simulink model "kamerol"  (R2021b)
settings: Solver=VariableStepAuto  StartTime=0.0  StopTime=10.0  RelTol=1e-3
undefined symbols (not defined in the file): admireDB
libraries: simulink_extras x104, simulink x24, sharedutil x1
(part 11 of 14)

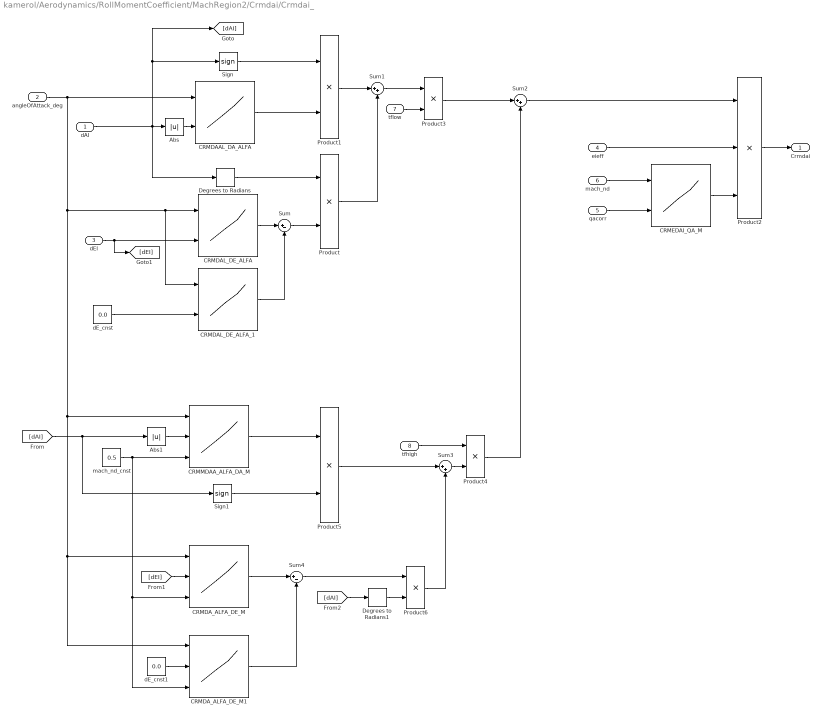
== system kamerol/Aerodynamics/RollMomentCoefficient/MachRegion2/Crmdai/Crmdai_ ==
  dAI : Inport
  angleOfAttack_deg : Inport  Port=2
  dEI : Inport  Port=3
  eieff : Inport  Port=4
  qacorr : Inport  Port=5
  mach_nd : Inport  Port=6
  tflow : Inport  Port=7
  tfhigh : Inport  Port=8
  Abs : Abs
  Abs1 : Abs
  CRMDAAL_DA_ALFA : Lookup_n-D  BreakpointsForDimension1=admireDB.aerodata_asym_ext.CRMDAAL.breakpoints.ALFA  BreakpointsForDimension2=admireDB.aerodata_asym_ext.CRMDAAL.breakpoints.DA  BreakpointsForDimension3=[5, 7]  Table=admireDB.aerodata_asym_ext.CRMDAAL.newTable  ExtrapMethod=Clip  InternalRulePriority=Speed  RndMeth=Simplest  InputSameDT=on
      settings: InputPortMap=u0,u1
  CRMDAL_DE_ALFA : Lookup_n-D  BreakpointsForDimension1=admireDB.aerodata_asym_ext.CRMDAL.breakpoints.ALFA  BreakpointsForDimension2=admireDB.aerodata_asym_ext.CRMDAL.breakpoints.DE  BreakpointsForDimension3=[5, 7]  Table=admireDB.aerodata_asym_ext.CRMDAL.newTable  ExtrapMethod=Clip  InternalRulePriority=Speed  RndMeth=Simplest  InputSameDT=on
      settings: InputPortMap=u0,u1
  CRMDAL_DE_ALFA_1 : Lookup_n-D  BreakpointsForDimension1=admireDB.aerodata_asym_ext.CRMDAL.breakpoints.ALFA  BreakpointsForDimension2=admireDB.aerodata_asym_ext.CRMDAL.breakpoints.DE  BreakpointsForDimension3=[5, 7]  Table=admireDB.aerodata_asym_ext.CRMDAL.newTable  ExtrapMethod=Clip  InternalRulePriority=Speed  RndMeth=Simplest  InputSameDT=on
      settings: InputPortMap=u0,u1
  CRMDA_ALFA_DE_M : Lookup_n-D  NumberOfTableDimensions=3  BreakpointsForDimension1=admireDB.aerodata_asym_ext.CRMDA.breakpoints.ALFA  BreakpointsForDimension2=admireDB.aerodata_asym_ext.CRMDA.breakpoints.DE  BreakpointsForDimension3=admireDB.aerodata_asym_ext.CRMDA.breakpoints.M  Table=admireDB.aerodata_asym_ext.CRMDA.newTable  ExtrapMethod=Clip  InternalRulePriority=Speed  RndMeth=Simplest  InputSameDT=on
      settings: InputPortMap=u0,u1,u2
  CRMDA_ALFA_DE_M1 : Lookup_n-D  NumberOfTableDimensions=3  BreakpointsForDimension1=admireDB.aerodata_asym_ext.CRMDA.breakpoints.ALFA  BreakpointsForDimension2=admireDB.aerodata_asym_ext.CRMDA.breakpoints.DE  BreakpointsForDimension3=admireDB.aerodata_asym_ext.CRMDA.breakpoints.M  Table=admireDB.aerodata_asym_ext.CRMDA.newTable  ExtrapMethod=Clip  InternalRulePriority=Speed  RndMeth=Simplest  InputSameDT=on
      settings: InputPortMap=u0,u1,u2
  CRMEDAI_QA_M : Lookup_n-D  BreakpointsForDimension1=admireDB.aerodata_asym_ext.CRMEDAI.breakpoints.M  BreakpointsForDimension2=admireDB.aerodata_asym_ext.CRMEDAI.breakpoints.QA  BreakpointsForDimension3=[5, 7]  Table=admireDB.aerodata_asym_ext.CRMEDAI.newTable  ExtrapMethod=Clip  InternalRulePriority=Speed  RndMeth=Simplest  InputSameDT=on
      settings: InputPortMap=u0,u1
  CRMMDAA_ALFA_DA_M : Lookup_n-D  NumberOfTableDimensions=3  BreakpointsForDimension1=admireDB.aerodata_asym_ext.CRMMDAA.breakpoints.ALFA  BreakpointsForDimension2=admireDB.aerodata_asym_ext.CRMMDAA.breakpoints.DA  BreakpointsForDimension3=admireDB.aerodata_asym_ext.CRMMDAA.breakpoints.M  Table=admireDB.aerodata_asym_ext.CRMMDAA.newTable  ExtrapMethod=Clip  InternalRulePriority=Speed  RndMeth=Simplest  InputSameDT=on
      settings: InputPortMap=u0,u1,u2
  Degrees to Radians : simulink_extras/Transformations/Degrees to Radians
  Degrees to Radians1 : simulink_extras/Transformations/Degrees to Radians
  Product{,1,3..4,6} (5 alike) : Product
  Product2 : Product  Inputs=3
  Product5 : Product  Inputs=**
  Sign : Signum
  Sign1 : Signum
  Sum : Sum  Inputs=|+-
  Sum1 : Sum  Inputs=|++
  Sum2 : Sum  Inputs=|++
  Sum3 : Sum  Inputs=|++
  Sum4 : Sum  Inputs=|+-
  dE_cnst : Constant  Value=0.0
  dE_cnst1 : Constant  Value=0.0
  mach_nd_cnst : Constant  Value=0.5
  Crmdai : Outport
  wires:
  Sum3/1 -> Product4/2
  Product6/1 -> Sum3/2
  [dAI] -> Degrees to Radians1/1
  Degrees to Radians1/1 -> Product6/2
  Sum4/1 -> Product6/1
  CRMDA_ALFA_DE_M1/1 -> Sum4/2
  CRMDA_ALFA_DE_M/1 -> Sum4/1
  dE_cnst1/1 -> CRMDA_ALFA_DE_M1/2
  [dEI] -> CRMDA_ALFA_DE_M/2
  mach_nd_cnst/1 -> CRMDA_ALFA_DE_M/3, CRMDA_ALFA_DE_M1/3, CRMMDAA_ALFA_DA_M/3
  Product5/1 -> Sum3/1
  Abs1/1 -> CRMMDAA_ALFA_DA_M/2
  CRMMDAA_ALFA_DA_M/1 -> Product5/1
  [dAI] -> Sign1/1, Abs1/1
  Sign1/1 -> Product5/2
  angleOfAttack_deg/1 -> CRMDAAL_DA_ALFA/1, CRMDAL_DE_ALFA/1, CRMDAL_DE_ALFA_1/1, CRMMDAA_ALFA_DA_M/1, CRMDA_ALFA_DE_M1/1, CRMDA_ALFA_DE_M/1
  Product4/1 -> Sum2/2
  Product3/1 -> Sum2/1
  tfhigh/1 -> Product4/1
  Sum2/1 -> Product2/1
  tflow/1 -> Product3/2
  Product2/1 -> Crmdai/1
  dAI/1 -> Sign/1, [dAI], Abs/1, Degrees to Radians/1
  Abs/1 -> CRMDAAL_DA_ALFA/2
  dE_cnst/1 -> CRMDAL_DE_ALFA_1/2
  dEI/1 -> [dEI], CRMDAL_DE_ALFA/2
  CRMDAL_DE_ALFA/1 -> Sum/1
  CRMDAL_DE_ALFA_1/1 -> Sum/2
  Sum/1 -> Product/2
  Degrees to Radians/1 -> Product/1
  CRMDAAL_DA_ALFA/1 -> Product1/2
  Sign/1 -> Product1/1
  Product1/1 -> Sum1/1
  Product/1 -> Sum1/2
  Sum1/1 -> Product3/1
  eieff/1 -> Product2/2
  qacorr/1 -> CRMEDAI_QA_M/2
  mach_nd/1 -> CRMEDAI_QA_M/1
  CRMEDAI_QA_M/1 -> Product2/3

== system kamerol/Aerodynamics/RollMomentCoefficient/MachRegion2/Crmdaib/Crmdaib_ ==
  angleOfAttack_deg : Inport
  dAI : Inport  Port=2
  angleOfSideslip_deg : Inport  Port=3
  eieff : Inport  Port=4
  tflow : Inport  Port=5
  Abs : Abs
  Abs1 : Abs
  Abs2 : Abs
  CRMDABAL_ALFA : Lookup_n-D  NumberOfTableDimensions=1  BreakpointsForDimension1=admireDB.aerodata_asym_ext.CRMDABAL.breakpoints.ALFA  BreakpointsForDimension3=[5, 7]  Table=admireDB.aerodata_asym_ext.CRMDABAL.newTable  ExtrapMethod=Clip  InternalRulePriority=Speed  RndMeth=Simplest  InputSameDT=on
  Constant : Constant  Value=1/30
  Constant1 : Constant  Value=1/20
  Product : Product  Inputs=*******
  Crmdaib : Outport
  wires:
  tflow/1 -> Product/7
  Product/1 -> Crmdaib/1
  angleOfAttack_deg/1 -> Abs/1
  CRMDABAL_ALFA/1 -> Product/1
  dAI/1 -> Abs1/1
  Abs/1 -> CRMDABAL_ALFA/1
  Abs1/1 -> Product/2
  Constant/1 -> Product/3
  angleOfSideslip_deg/1 -> Abs2/1
  Constant1/1 -> Product/5
  Abs2/1 -> Product/4
  eieff/1 -> Product/6

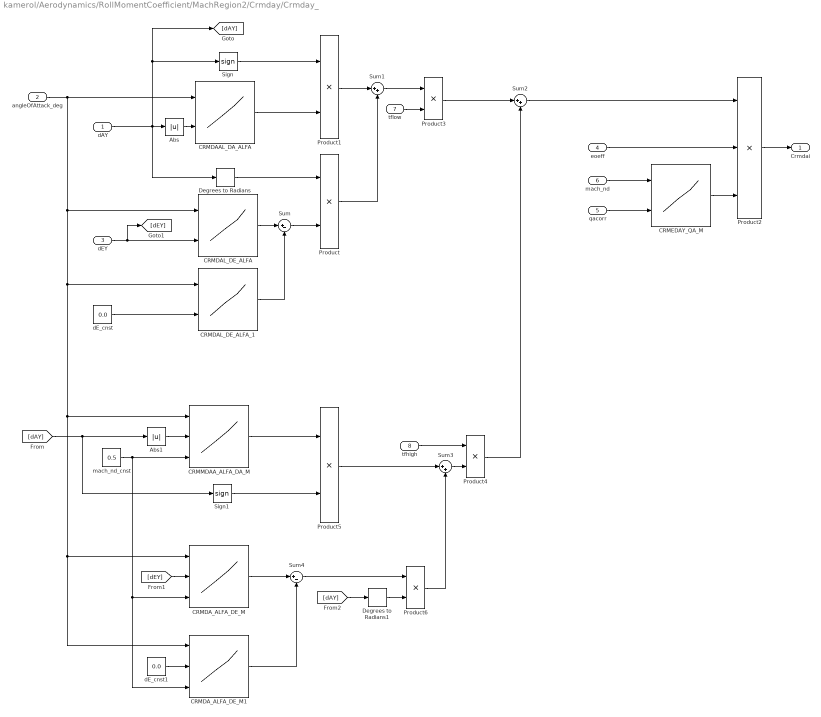
== system kamerol/Aerodynamics/RollMomentCoefficient/MachRegion2/Crmday/Crmday_ ==
  dAY : Inport
  angleOfAttack_deg : Inport  Port=2
  dEY : Inport  Port=3
  eoeff : Inport  Port=4
  qacorr : Inport  Port=5
  mach_nd : Inport  Port=6
  tflow : Inport  Port=7
  tfhigh : Inport  Port=8
  Abs : Abs
  Abs1 : Abs
  CRMDAAL_DA_ALFA : Lookup_n-D  BreakpointsForDimension1=admireDB.aerodata_asym_ext.CRMDAAL.breakpoints.ALFA  BreakpointsForDimension2=admireDB.aerodata_asym_ext.CRMDAAL.breakpoints.DA  BreakpointsForDimension3=[5, 7]  Table=admireDB.aerodata_asym_ext.CRMDAAL.newTable  ExtrapMethod=Clip  InternalRulePriority=Speed  RndMeth=Simplest  InputSameDT=on
      settings: InputPortMap=u0,u1
  CRMDAL_DE_ALFA : Lookup_n-D  BreakpointsForDimension1=admireDB.aerodata_asym_ext.CRMDAL.breakpoints.ALFA  BreakpointsForDimension2=admireDB.aerodata_asym_ext.CRMDAL.breakpoints.DE  BreakpointsForDimension3=[5, 7]  Table=admireDB.aerodata_asym_ext.CRMDAL.newTable  ExtrapMethod=Clip  InternalRulePriority=Speed  RndMeth=Simplest  InputSameDT=on
      settings: InputPortMap=u0,u1
  CRMDAL_DE_ALFA_1 : Lookup_n-D  BreakpointsForDimension1=admireDB.aerodata_asym_ext.CRMDAL.breakpoints.ALFA  BreakpointsForDimension2=admireDB.aerodata_asym_ext.CRMDAL.breakpoints.DE  BreakpointsForDimension3=[5, 7]  Table=admireDB.aerodata_asym_ext.CRMDAL.newTable  ExtrapMethod=Clip  InternalRulePriority=Speed  RndMeth=Simplest  InputSameDT=on
      settings: InputPortMap=u0,u1
  CRMDA_ALFA_DE_M : Lookup_n-D  NumberOfTableDimensions=3  BreakpointsForDimension1=admireDB.aerodata_asym_ext.CRMDA.breakpoints.ALFA  BreakpointsForDimension2=admireDB.aerodata_asym_ext.CRMDA.breakpoints.DE  BreakpointsForDimension3=admireDB.aerodata_asym_ext.CRMDA.breakpoints.M  Table=admireDB.aerodata_asym_ext.CRMDA.newTable  ExtrapMethod=Clip  InternalRulePriority=Speed  RndMeth=Simplest  InputSameDT=on
      settings: InputPortMap=u0,u1,u2
  CRMDA_ALFA_DE_M1 : Lookup_n-D  NumberOfTableDimensions=3  BreakpointsForDimension1=admireDB.aerodata_asym_ext.CRMDA.breakpoints.ALFA  BreakpointsForDimension2=admireDB.aerodata_asym_ext.CRMDA.breakpoints.DE  BreakpointsForDimension3=admireDB.aerodata_asym_ext.CRMDA.breakpoints.M  Table=admireDB.aerodata_asym_ext.CRMDA.newTable  ExtrapMethod=Clip  InternalRulePriority=Speed  RndMeth=Simplest  InputSameDT=on
      settings: InputPortMap=u0,u1,u2
  CRMEDAY_QA_M : Lookup_n-D  BreakpointsForDimension1=admireDB.aerodata_asym_ext.CRMEDAY.breakpoints.M  BreakpointsForDimension2=admireDB.aerodata_asym_ext.CRMEDAY.breakpoints.QA  BreakpointsForDimension3=[5, 7]  Table=admireDB.aerodata_asym_ext.CRMEDAY.newTable  ExtrapMethod=Clip  InternalRulePriority=Speed  RndMeth=Simplest  InputSameDT=on
      settings: InputPortMap=u0,u1
  CRMMDAA_ALFA_DA_M : Lookup_n-D  NumberOfTableDimensions=3  BreakpointsForDimension1=admireDB.aerodata_asym_ext.CRMMDAA.breakpoints.ALFA  BreakpointsForDimension2=admireDB.aerodata_asym_ext.CRMMDAA.breakpoints.DA  BreakpointsForDimension3=admireDB.aerodata_asym_ext.CRMMDAA.breakpoints.M  Table=admireDB.aerodata_asym_ext.CRMMDAA.newTable  ExtrapMethod=Clip  InternalRulePriority=Speed  RndMeth=Simplest  InputSameDT=on
      settings: InputPortMap=u0,u1,u2
  Degrees to Radians : simulink_extras/Transformations/Degrees to Radians
  Degrees to Radians1 : simulink_extras/Transformations/Degrees to Radians
  Product{,1,3..4,6} (5 alike) : Product
  Product2 : Product  Inputs=3
  Product5 : Product  Inputs=**
  Sign : Signum
  Sign1 : Signum
  Sum : Sum  Inputs=|+-
  Sum1 : Sum  Inputs=|++
  Sum2 : Sum  Inputs=|++
  Sum3 : Sum  Inputs=|++
  Sum4 : Sum  Inputs=|+-
  dE_cnst : Constant  Value=0.0
  dE_cnst1 : Constant  Value=0.0
  mach_nd_cnst : Constant  Value=0.5
  Crmdai : Outport
  wires:
  Sum3/1 -> Product4/2
  Product6/1 -> Sum3/2
  [dAY] -> Degrees to Radians1/1
  Degrees to Radians1/1 -> Product6/2
  Sum4/1 -> Product6/1
  CRMDA_ALFA_DE_M1/1 -> Sum4/2
  CRMDA_ALFA_DE_M/1 -> Sum4/1
  dE_cnst1/1 -> CRMDA_ALFA_DE_M1/2
  [dEY] -> CRMDA_ALFA_DE_M/2
  mach_nd_cnst/1 -> CRMDA_ALFA_DE_M/3, CRMDA_ALFA_DE_M1/3, CRMMDAA_ALFA_DA_M/3
  Product5/1 -> Sum3/1
  Abs1/1 -> CRMMDAA_ALFA_DA_M/2
  CRMMDAA_ALFA_DA_M/1 -> Product5/1
  [dAY] -> Sign1/1, Abs1/1
  Sign1/1 -> Product5/2
  angleOfAttack_deg/1 -> CRMDAAL_DA_ALFA/1, CRMDAL_DE_ALFA/1, CRMMDAA_ALFA_DA_M/1, CRMDA_ALFA_DE_M1/1, CRMDA_ALFA_DE_M/1, CRMDAL_DE_ALFA_1/1
  Product4/1 -> Sum2/2
  Product3/1 -> Sum2/1
  tfhigh/1 -> Product4/1
  Sum2/1 -> Product2/1
  tflow/1 -> Product3/2
  Product2/1 -> Crmdai/1
  dAY/1 -> Sign/1, [dAY], Abs/1, Degrees to Radians/1
  Abs/1 -> CRMDAAL_DA_ALFA/2
  dE_cnst/1 -> CRMDAL_DE_ALFA_1/2
  dEY/1 -> CRMDAL_DE_ALFA/2, [dEY]
  CRMDAL_DE_ALFA/1 -> Sum/1
  CRMDAL_DE_ALFA_1/1 -> Sum/2
  Sum/1 -> Product/2
  Degrees to Radians/1 -> Product/1
  CRMDAAL_DA_ALFA/1 -> Product1/2
  Sign/1 -> Product1/1
  Product1/1 -> Sum1/1
  Product/1 -> Sum1/2
  Sum1/1 -> Product3/1
  eoeff/1 -> Product2/2
  qacorr/1 -> CRMEDAY_QA_M/2
  mach_nd/1 -> CRMEDAY_QA_M/1
  CRMEDAY_QA_M/1 -> Product2/3

== system kamerol/Aerodynamics/RollMomentCoefficient/MachRegion2/Crmdayb/Crmdayb_ ==
  angleOfAttack_deg : Inport
  dAY : Inport  Port=2
  angleOfSideslip_deg : Inport  Port=3
  eoeff : Inport  Port=4
  tflow : Inport  Port=5
  Abs : Abs
  Abs1 : Abs
  Abs2 : Abs
  CRMDABAL_ALFA : Lookup_n-D  NumberOfTableDimensions=1  BreakpointsForDimension1=admireDB.aerodata_asym_ext.CRMDABAL.breakpoints.ALFA  BreakpointsForDimension3=[5, 7]  Table=admireDB.aerodata_asym_ext.CRMDABAL.newTable  ExtrapMethod=Clip  InternalRulePriority=Speed  RndMeth=Simplest  InputSameDT=on
  Constant : Constant  Value=1/30
  Constant1 : Constant  Value=1/20
  Product : Product  Inputs=*******
  Crmdayb : Outport
  wires:
  tflow/1 -> Product/7
  eoeff/1 -> Product/6
  Abs2/1 -> Product/4
  Constant1/1 -> Product/5
  angleOfSideslip_deg/1 -> Abs2/1
  Constant/1 -> Product/3
  Abs1/1 -> Product/2
  Abs/1 -> CRMDABAL_ALFA/1
  dAY/1 -> Abs1/1
  CRMDABAL_ALFA/1 -> Product/1
  angleOfAttack_deg/1 -> Abs/1
  Product/1 -> Crmdayb/1

== system kamerol/Aerodynamics/RollMomentCoefficient/MachRegion2/Crmdna/Crmdna_ ==
  dNE : Inport
  angleOfAttack_deg : Inport  Port=2
  tflow : Inport  Port=3
  tfhigh : Inport  Port=4
  dNA : Inport  Port=5
  CRMDNAAL_DNE_ALFA : Lookup_n-D  BreakpointsForDimension1=admireDB.aerodata_asym_ext.CRMDNAAL.breakpoints.ALFA  BreakpointsForDimension2=admireDB.aerodata_asym_ext.CRMDNAAL.breakpoints.DNE  BreakpointsForDimension3=[5, 7]  Table=admireDB.aerodata_asym_ext.CRMDNAAL.newTable  ExtrapMethod=Clip  InternalRulePriority=Speed  RndMeth=Simplest  InputSameDT=on
      settings: InputPortMap=u0,u1
  CRMDNAAM_ALFA_M : Lookup_n-D  BreakpointsForDimension1=admireDB.aerodata_asym_ext.CRMDNAAM.breakpoints.M  BreakpointsForDimension2=admireDB.aerodata_asym_ext.CRMDNAAM.breakpoints.ALFA  BreakpointsForDimension3=[5, 7]  Table=admireDB.aerodata_asym_ext.CRMDNAAM.newTable  ExtrapMethod=Clip  InternalRulePriority=Speed  RndMeth=Simplest  InputSameDT=on
      settings: InputPortMap=u0,u1
  Degrees to Radians : simulink_extras/Transformations/Degrees to Radians
  Product : Product  Inputs=**
  Product1 : Product
  Product2 : Product  Inputs=**
  Sum : Sum  Inputs=|++
  mach_nd_cnst : Constant  Value=0.5
  Crmdna : Outport
  wires:
  Sum/1 -> Product/1
  Product2/1 -> Sum/2
  Product1/1 -> Sum/1
  CRMDNAAM_ALFA_M/1 -> Product2/1
  tfhigh/1 -> Product2/2
  mach_nd_cnst/1 -> CRMDNAAM_ALFA_M/1
  tflow/1 -> Product1/2
  Product/1 -> Crmdna/1
  angleOfAttack_deg/1 -> CRMDNAAL_DNE_ALFA/1, CRMDNAAM_ALFA_M/2
  dNE/1 -> CRMDNAAL_DNE_ALFA/2
  dNA/1 -> Degrees to Radians/1
  CRMDNAAL_DNE_ALFA/1 -> Product1/1
  Degrees to Radians/1 -> Product/2

== system kamerol/Aerodynamics/RollMomentCoefficient/MachRegion2/Crmdr/Crmdr_ ==
  angleOfAttack_deg : Inport
  dR : Inport  Port=2
  tfhigh : Inport  Port=3
  angleOfSideslip_deg : Inport  Port=4
  tflow : Inport  Port=5
  qacorr : Inport  Port=6
  mach_nd : Inport  Port=7
  Abs : Abs
  CRMBDRAL_ALFA_DR_BETA : Lookup_n-D  NumberOfTableDimensions=3  BreakpointsForDimension1=admireDB.aerodata_asym_ext.CRMBDRAL.breakpoints.ALFA  BreakpointsForDimension2=admireDB.aerodata_asym_ext.CRMBDRAL.breakpoints.DR  BreakpointsForDimension3=admireDB.aerodata_asym_ext.CRMBDRAL.breakpoints.BETA  Table=admireDB.aerodata_asym_ext.CRMBDRAL.newTable  ExtrapMethod=Clip  InternalRulePriority=Speed  RndMeth=Simplest  InputSameDT=on
      settings: InputPortMap=u0,u1,u2
  CRMDRM_M : Lookup_n-D  NumberOfTableDimensions=1  BreakpointsForDimension1=admireDB.aerodata_asym_ext.CRMDRM.breakpoints.M  BreakpointsForDimension3=[5, 7]  Table=admireDB.aerodata_asym_ext.CRMDRM.newTable  ExtrapMethod=Clip  InternalRulePriority=Speed  RndMeth=Simplest  InputSameDT=on
  CRMEDR_QA_M : Lookup_n-D  BreakpointsForDimension1=admireDB.aerodata_asym_ext.CRMEDR.breakpoints.M  BreakpointsForDimension2=admireDB.aerodata_asym_ext.CRMEDR.breakpoints.QA  BreakpointsForDimension3=[5, 7]  Table=admireDB.aerodata_asym_ext.CRMEDR.newTable  ExtrapMethod=Clip  InternalRulePriority=Speed  RndMeth=Simplest  InputSameDT=on
      settings: InputPortMap=u0,u1
  Degrees to Radians : simulink_extras/Transformations/Degrees to Radians
  Product : Product
  Product1 : Product  Inputs=***
  Product2 : Product
  Sum : Sum  Inputs=++|
  mach_nd_cnst : Constant  Value=0.5
  Crmdr : Outport
  wires:
  Abs/1 -> CRMBDRAL_ALFA_DR_BETA/3
  Product2/1 -> Crmdr/1
  CRMEDR_QA_M/1 -> Product2/2
  Sum/1 -> Product2/1
  Product1/1 -> Sum/2
  CRMDRM_M/1 -> Product1/1
  Degrees to Radians/1 -> Product1/2
  mach_nd_cnst/1 -> CRMDRM_M/1
  tfhigh/1 -> Product1/3
  dR/1 -> Degrees to Radians/1, CRMBDRAL_ALFA_DR_BETA/2
  Product/1 -> Sum/1
  qacorr/1 -> CRMEDR_QA_M/2
  mach_nd/1 -> CRMEDR_QA_M/1
  angleOfSideslip_deg/1 -> Abs/1
  angleOfAttack_deg/1 -> CRMBDRAL_ALFA_DR_BETA/1
  tflow/1 -> Product/2
  CRMBDRAL_ALFA_DR_BETA/1 -> Product/1

== system kamerol/Aerodynamics/RollMomentCoefficient/MachRegion2/Crmp/Crmp_ ==
  dN : Inport
  angleOfAttack_deg : Inport  Port=2
  qacorr : Inport  Port=3
  mach_nd : Inport  Port=4
  pc : Inport  Port=5
  tflow : Inport  Port=6
  tfhigh : Inport  Port=7
  CRMEP_QA_M : Lookup_n-D  BreakpointsForDimension1=admireDB.aerodata_asym_ext.CRMEP.breakpoints.M  BreakpointsForDimension2=admireDB.aerodata_asym_ext.CRMEP.breakpoints.QA  BreakpointsForDimension3=[5, 7]  Table=admireDB.aerodata_asym_ext.CRMEP.newTable  ExtrapMethod=Clip  InternalRulePriority=Speed  RndMeth=Simplest  InputSameDT=on
      settings: InputPortMap=u0,u1
  CRMPAL_DN_ALFA : Lookup_n-D  BreakpointsForDimension1=admireDB.aerodata_asym_ext.CRMPAL.breakpoints.ALFA  BreakpointsForDimension2=admireDB.aerodata_asym_ext.CRMPAL.breakpoints.DN  BreakpointsForDimension3=[5, 7]  Table=admireDB.aerodata_asym_ext.CRMPAL.newTable  ExtrapMethod=Clip  InternalRulePriority=Speed  RndMeth=Simplest  InputSameDT=on
      settings: InputPortMap=u0,u1
  CRMPAM_ALFA_M : Lookup_n-D  BreakpointsForDimension1=admireDB.aerodata_asym_ext.CRMPAM.breakpoints.M  BreakpointsForDimension2=admireDB.aerodata_asym_ext.CRMPAM.breakpoints.ALFA  BreakpointsForDimension3=[5, 7]  Table=admireDB.aerodata_asym_ext.CRMPAM.newTable  ExtrapMethod=Clip  InternalRulePriority=Speed  RndMeth=Simplest  InputSameDT=on
      settings: InputPortMap=u0,u1
  Product : Product  Inputs=3
  Product1 : Product  Inputs=**
  Product2 : Product  Inputs=**
  Sum : Sum  Inputs=|++
  mach_nd_cnst : Constant  Value=0.5
  Crmp : Outport
  wires:
  Sum/1 -> Product/1
  Product2/1 -> Sum/2
  Product1/1 -> Sum/1
  tfhigh/1 -> Product2/1
  CRMPAM_ALFA_M/1 -> Product2/2
  tflow/1 -> Product1/2
  mach_nd_cnst/1 -> CRMPAM_ALFA_M/1
  qacorr/1 -> CRMEP_QA_M/2
  mach_nd/1 -> CRMEP_QA_M/1
  angleOfAttack_deg/1 -> CRMPAL_DN_ALFA/1, CRMPAM_ALFA_M/2
  dN/1 -> CRMPAL_DN_ALFA/2
  CRMPAL_DN_ALFA/1 -> Product1/1
  CRMEP_QA_M/1 -> Product/3
  pc/1 -> Product/2
  Product/1 -> Crmp/1

== system kamerol/Aerodynamics/RollMomentCoefficient/MachRegion2/Crmpbeta/Crmpbeta_ ==
  angleOfSideslip_deg : Inport
  pc : Inport  Port=2
  angleOfAttack_deg : Inport  Port=3
  tflow : Inport  Port=4
  Abs : Abs
  CRMPBA_BETA_ALFA : Lookup_n-D  BreakpointsForDimension1=admireDB.aerodata_asym_ext.CRMPBA.breakpoints.ALFA  BreakpointsForDimension2=admireDB.aerodata_asym_ext.CRMPBA.breakpoints.BETA  BreakpointsForDimension3=[5, 7]  Table=admireDB.aerodata_asym_ext.CRMPBA.newTable  ExtrapMethod=Clip  InternalRulePriority=Speed  RndMeth=Simplest  InputSameDT=on
      settings: InputPortMap=u0,u1
  Product : Product  Inputs=***
  Crmpbeta : Outport
  wires:
  tflow/1 -> Product/3
  Product/1 -> Crmpbeta/1
  pc/1 -> Product/2
  angleOfAttack_deg/1 -> CRMPBA_BETA_ALFA/1
  angleOfSideslip_deg/1 -> Abs/1
  CRMPBA_BETA_ALFA/1 -> Product/1
  Abs/1 -> CRMPBA_BETA_ALFA/2

== system kamerol/Aerodynamics/RollMomentCoefficient/MachRegion2/Crmr/Crmr_ ==
  dN : Inport
  angleOfAttack_deg : Inport  Port=2
  rc : Inport  Port=3
  tflow : Inport  Port=4
  tfhigh : Inport  Port=5
  CRMRAL_DN_ALFA : Lookup_n-D  BreakpointsForDimension1=admireDB.aerodata_asym_ext.CRMRAL.breakpoints.ALFA  BreakpointsForDimension2=admireDB.aerodata_asym_ext.CRMRAL.breakpoints.DN  BreakpointsForDimension3=[5, 7]  Table=admireDB.aerodata_asym_ext.CRMRAL.newTable  ExtrapMethod=Clip  InternalRulePriority=Speed  RndMeth=Simplest  InputSameDT=on
      settings: InputPortMap=u0,u1
  CRMRAM_ALFA_M : Lookup_n-D  BreakpointsForDimension1=admireDB.aerodata_asym_ext.CRMRAM.breakpoints.M  BreakpointsForDimension2=admireDB.aerodata_asym_ext.CRMRAM.breakpoints.ALFA  BreakpointsForDimension3=[5, 7]  Table=admireDB.aerodata_asym_ext.CRMRAM.newTable  ExtrapMethod=Clip  InternalRulePriority=Speed  RndMeth=Simplest  InputSameDT=on
      settings: InputPortMap=u0,u1
  Product : Product  Inputs=**
  Product1 : Product  Inputs=**
  Product2 : Product  Inputs=**
  Sum : Sum  Inputs=|++
  mach_nd_cnst : Constant  Value=0.5
  Crmr : Outport
  wires:
  Sum/1 -> Product/1
  Product2/1 -> Sum/2
  Product1/1 -> Sum/1
  CRMRAM_ALFA_M/1 -> Product2/2
  tfhigh/1 -> Product2/1
  tflow/1 -> Product1/2
  mach_nd_cnst/1 -> CRMRAM_ALFA_M/1
  rc/1 -> Product/2
  Product/1 -> Crmr/1
  angleOfAttack_deg/1 -> CRMRAL_DN_ALFA/1, CRMRAM_ALFA_M/2
  dN/1 -> CRMRAL_DN_ALFA/2
  CRMRAL_DN_ALFA/1 -> Product1/1

== system kamerol/Aerodynamics/RollMomentCoefficient/MachRegion2/Crmrbeta/Crmrbeta_ ==
  angleOfSideslip_deg : Inport
  angleOfAttack_deg : Inport  Port=2
  rc : Inport  Port=3
  tflow : Inport  Port=4
  Abs : Abs
  CRMRBA_BETA_ALFA : Lookup_n-D  BreakpointsForDimension1=admireDB.aerodata_asym_ext.CRMRBA.breakpoints.ALFA  BreakpointsForDimension2=admireDB.aerodata_asym_ext.CRMRBA.breakpoints.BETA  BreakpointsForDimension3=[5, 7]  Table=admireDB.aerodata_asym_ext.CRMRBA.newTable  ExtrapMethod=Clip  InternalRulePriority=Speed  RndMeth=Simplest  InputSameDT=on
      settings: InputPortMap=u0,u1
  Product : Product  Inputs=***
  Crmrbeta : Outport
  wires:
  tflow/1 -> Product/3
  CRMRBA_BETA_ALFA/1 -> Product/1
  Product/1 -> Crmrbeta/1
  rc/1 -> Product/2
  angleOfAttack_deg/1 -> CRMRBA_BETA_ALFA/1
  angleOfSideslip_deg/1 -> Abs/1
  Abs/1 -> CRMRBA_BETA_ALFA/2

== system kamerol/Aerodynamics/RollMomentCoefficient/MachRegion2/Crmrde/Crmrde_ ==
  mach_nd : Inport
  angleOfAttack_deg : Inport  Port=2
  rc : Inport  Port=3
  dEI : Inport  Port=4
  eieff : Inport  Port=5
  dey : Inport  Port=6
  eoeff : Inport  Port=7
  Abs : Abs
  CRMRDEM_M : Lookup_n-D  NumberOfTableDimensions=1  BreakpointsForDimension1=admireDB.aerodata_asym_ext.CRMRDEM.breakpoints.M  BreakpointsForDimension3=[5, 7]  Table=admireDB.aerodata_asym_ext.CRMRDEM.newTable  ExtrapMethod=Clip  InternalRulePriority=Speed  RndMeth=Simplest  InputSameDT=on
  CRMRKA_ALFA : Lookup_n-D  NumberOfTableDimensions=1  BreakpointsForDimension1=admireDB.aerodata_asym_ext.CRMRKA.breakpoints.ALFA  BreakpointsForDimension3=[5, 7]  Table=admireDB.aerodata_asym_ext.CRMRKA.newTable  ExtrapMethod=Clip  InternalRulePriority=Speed  RndMeth=Simplest  InputSameDT=on
  Constant : Constant  Value=1/30
  Constant1 : Constant  Value=1/30
  Product : Product  Inputs=****
  Product1 : Product  Inputs=3
  Product2 : Product  Inputs=3
  Sum : Sum  Inputs=|++
  Crmrde : Outport
  wires:
  Abs/1 -> CRMRKA_ALFA/1
  rc/1 -> Product/3
  Product/1 -> Crmrde/1
  angleOfAttack_deg/1 -> Abs/1
  mach_nd/1 -> CRMRDEM_M/1
  CRMRDEM_M/1 -> Product/1
  CRMRKA_ALFA/1 -> Product/2
  dEI/1 -> Product1/1
  eieff/1 -> Product1/3
  Constant/1 -> Product1/2
  Constant1/1 -> Product2/2
  eoeff/1 -> Product2/3
  dey/1 -> Product2/1
  Product1/1 -> Sum/1
  Product2/1 -> Sum/2
  Sum/1 -> Product/4

== system kamerol/Aerodynamics/RollMomentCoefficient/MachRegion3/Crmbde/Crmbde_ ==
  angleOfAttack_deg : Inport
  dN : Inport  Port=2
  dEI : Inport  Port=3
  angleOfSideslip_deg : Inport  Port=4
  dEY : Inport  Port=5
  eieff : Inport  Port=6
  eoeff : Inport  Port=7
  mach_nd : Inport  Port=8
  Abs : Abs
  CRMBKM_M : Lookup_n-D  NumberOfTableDimensions=1  BreakpointsForDimension1=admireDB.aerodata_asym_ext.CRMBKM.breakpoints.M  BreakpointsForDimension3=[5, 7]  Table=admireDB.aerodata_asym_ext.CRMBKM.newTable  ExtrapMethod=Clip  InternalRulePriority=Speed  RndMeth=Simplest  InputSameDT=on
  CRMDEB_ALFA_DN_DE_BETA : Lookup_n-D  NumberOfTableDimensions=4  BreakpointsForDimension1=admireDB.aerodata_asym_ext.CRMDEB.breakpoints.ALFA  BreakpointsForDimension2=admireDB.aerodata_asym_ext.CRMDEB.breakpoints.DN  BreakpointsForDimension3=admireDB.aerodata_asym_ext.CRMDEB.breakpoints.DE  BreakpointsForDimension4=admireDB.aerodata_asym_ext.CRMDEB.breakpoints.BETA  Table=admireDB.aerodata_asym_ext.CRMDEB.newTable  ExtrapMethod=Clip  InternalRulePriority=Speed  RndMeth=Simplest  InputSameDT=on
      settings: InputPortMap=u0,u1,u2,u3
  CRMDEB_ALFA_DN_DE_BETA1 : Lookup_n-D  NumberOfTableDimensions=4  BreakpointsForDimension1=admireDB.aerodata_asym_ext.CRMDEB.breakpoints.ALFA  BreakpointsForDimension2=admireDB.aerodata_asym_ext.CRMDEB.breakpoints.DN  BreakpointsForDimension3=admireDB.aerodata_asym_ext.CRMDEB.breakpoints.DE  BreakpointsForDimension4=admireDB.aerodata_asym_ext.CRMDEB.breakpoints.BETA  Table=admireDB.aerodata_asym_ext.CRMDEB.newTable  ExtrapMethod=Clip  InternalRulePriority=Speed  RndMeth=Simplest  InputSameDT=on
      settings: InputPortMap=u0,u1,u2,u3
  Product : Product  Inputs=**
  Product1 : Product  Inputs=**
  Product2 : Product  Inputs=3
  Sign : Signum
  Sum : Sum  Inputs=|++
  Crmbde : Outport
  wires:
  dEY/1 -> CRMDEB_ALFA_DN_DE_BETA1/3
  angleOfAttack_deg/1 -> CRMDEB_ALFA_DN_DE_BETA/1, CRMDEB_ALFA_DN_DE_BETA1/1
  dN/1 -> CRMDEB_ALFA_DN_DE_BETA/2, CRMDEB_ALFA_DN_DE_BETA1/2
  dEI/1 -> CRMDEB_ALFA_DN_DE_BETA/3
  Abs/1 -> CRMDEB_ALFA_DN_DE_BETA/4, CRMDEB_ALFA_DN_DE_BETA1/4
  CRMBKM_M/1 -> Product2/3
  mach_nd/1 -> CRMBKM_M/1
  Sign/1 -> Product2/1
  Product2/1 -> Crmbde/1
  Product1/1 -> Sum/2
  Product/1 -> Sum/1
  Sum/1 -> Product2/2
  eoeff/1 -> Product1/1
  eieff/1 -> Product/2
  CRMDEB_ALFA_DN_DE_BETA1/1 -> Product1/2
  CRMDEB_ALFA_DN_DE_BETA/1 -> Product/1
  angleOfSideslip_deg/1 -> Sign/1, Abs/1

== system kamerol/Aerodynamics/RollMomentCoefficient/MachRegion3/Crmbdle/Crmbdle_ ==
  angleOfAttack_deg : Inport
  dEI : Inport  Port=2
  mach_nd : Inport  Port=3
  dEY : Inport  Port=4
  eieff : Inport  Port=5
  eoeff : Inport  Port=6
  angleOfSideslip_deg : Inport  Port=7
  dLE : Inport  Port=8
  CRMBDLE_ALFA_DE_M : Lookup_n-D  NumberOfTableDimensions=3  BreakpointsForDimension1=admireDB.aerodata_asym_ext.CRMBDLE.breakpoints.ALFA  BreakpointsForDimension2=admireDB.aerodata_asym_ext.CRMBDLE.breakpoints.DE  BreakpointsForDimension3=admireDB.aerodata_asym_ext.CRMBDLE.breakpoints.M  Table=admireDB.aerodata_asym_ext.CRMBDLE.newTable  ExtrapMethod=Clip  InternalRulePriority=Speed  RndMeth=Simplest  InputSameDT=on
      settings: InputPortMap=u0,u1,u2
  CRMBDLE_ALFA_DE_M1 : Lookup_n-D  NumberOfTableDimensions=3  BreakpointsForDimension1=admireDB.aerodata_asym_ext.CRMBDLE.breakpoints.ALFA  BreakpointsForDimension2=admireDB.aerodata_asym_ext.CRMBDLE.breakpoints.DE  BreakpointsForDimension3=admireDB.aerodata_asym_ext.CRMBDLE.breakpoints.M  Table=admireDB.aerodata_asym_ext.CRMBDLE.newTable  ExtrapMethod=Clip  InternalRulePriority=Speed  RndMeth=Simplest  InputSameDT=on
      settings: InputPortMap=u0,u1,u2
  Constant : Constant  Value=1/27
  Degrees to Radians : simulink_extras/Transformations/Degrees to Radians
  Product : Product  Inputs=**
  Product1 : Product  Inputs=**
  Product2 : Product  Inputs=****
  Sum : Sum  Inputs=|++
  Crmbdle : Outport
  wires:
  dEY/1 -> CRMBDLE_ALFA_DE_M1/2
  dEI/1 -> CRMBDLE_ALFA_DE_M/2
  mach_nd/1 -> CRMBDLE_ALFA_DE_M/3, CRMBDLE_ALFA_DE_M1/3
  angleOfAttack_deg/1 -> CRMBDLE_ALFA_DE_M/1, CRMBDLE_ALFA_DE_M1/1
  Product2/1 -> Crmbdle/1
  Constant/1 -> Product2/4
  Sum/1 -> Product2/2
  Product1/1 -> Sum/2
  Product/1 -> Sum/1
  dLE/1 -> Product2/3
  Degrees to Radians/1 -> Product2/1
  angleOfSideslip_deg/1 -> Degrees to Radians/1
  CRMBDLE_ALFA_DE_M1/1 -> Product1/1
  eoeff/1 -> Product1/2
  CRMBDLE_ALFA_DE_M/1 -> Product/1
  eieff/1 -> Product/2

== system kamerol/Aerodynamics/RollMomentCoefficient/MachRegion3/Crmbdn/Crmbdn_ ==
  dN : Inport
  mach_nd : Inport  Port=2
  angleOfSideslip_deg : Inport  Port=3
  CRMBMDN_DN_M : Lookup_n-D  BreakpointsForDimension1=admireDB.aerodata_asym_ext.CRMBMDN.breakpoints.M  BreakpointsForDimension2=admireDB.aerodata_asym_ext.CRMBMDN.breakpoints.DN  BreakpointsForDimension3=[5, 7]  Table=admireDB.aerodata_asym_ext.CRMBMDN.newTable  ExtrapMethod=Clip  InternalRulePriority=Speed  RndMeth=Simplest  InputSameDT=on
      settings: InputPortMap=u0,u1
  Degrees to Radians : simulink_extras/Transformations/Degrees to Radians
  Product : Product  Inputs=**
  Crmbdn : Outport
  wires:
  Product/1 -> Crmbdn/1
  CRMBMDN_DN_M/1 -> Product/1
  angleOfSideslip_deg/1 -> Degrees to Radians/1
  dN/1 -> CRMBMDN_DN_M/2
  Degrees to Radians/1 -> Product/2
  mach_nd/1 -> CRMBMDN_DN_M/1

== system kamerol/Aerodynamics/RollMomentCoefficient/MachRegion3/Crmbeta/Crmbeta_ ==
  mach_nd : Inport
  angleOfAttack_deg : Inport  Port=2
  angleOfSideslip_deg : Inport  Port=3
  qacorr : Inport  Port=4
  CRMBMA_M_ALFA : Lookup_n-D  BreakpointsForDimension1=admireDB.aerodata_asym_ext.CRMBMA.breakpoints.ALFA  BreakpointsForDimension2=admireDB.aerodata_asym_ext.CRMBMA.breakpoints.M  BreakpointsForDimension3=[5, 7]  Table=admireDB.aerodata_asym_ext.CRMBMA.newTable  ExtrapMethod=Clip  InternalRulePriority=Speed  RndMeth=Simplest  InputSameDT=on
      settings: InputPortMap=u0,u1
  CRMEB_QA_M : Lookup_n-D  BreakpointsForDimension1=admireDB.aerodata_asym_ext.CRMEB.breakpoints.M  BreakpointsForDimension2=admireDB.aerodata_asym_ext.CRMEB.breakpoints.QA  BreakpointsForDimension3=[5, 7]  Table=admireDB.aerodata_asym_ext.CRMEB.newTable  ExtrapMethod=Clip  InternalRulePriority=Speed  RndMeth=Simplest  InputSameDT=on
      settings: InputPortMap=u0,u1
  Degrees to Radians : simulink_extras/Transformations/Degrees to Radians
  Product1 : Product
  Sum : Sum  Inputs=|++
  Crmbeta : Outport
  wires:
  Product1/1 -> Crmbeta/1
  Sum/1 -> Product1/1
  CRMEB_QA_M/1 -> Sum/2
  Degrees to Radians/1 -> Product1/2
  angleOfSideslip_deg/1 -> Degrees to Radians/1
  qacorr/1 -> CRMEB_QA_M/2
  angleOfAttack_deg/1 -> CRMBMA_M_ALFA/1
  mach_nd/1 -> CRMBMA_M_ALFA/2, CRMEB_QA_M/1
  CRMBMA_M_ALFA/1 -> Sum/1

== system kamerol/Aerodynamics/RollMomentCoefficient/MachRegion3/Crmbetad/Crmbetad_ ==
  angleOfAttack_deg : Inport
  mach_nd : Inport  Port=2
  betad : Inport  Port=3
  CRMBDH_ALFA_M : Lookup_n-D  BreakpointsForDimension1=admireDB.aerodata_asym_ext.CRMBDH.breakpoints.M  BreakpointsForDimension2=admireDB.aerodata_asym_ext.CRMBDH.breakpoints.ALFA  BreakpointsForDimension3=[5, 7]  Table=admireDB.aerodata_asym_ext.CRMBDH.newTable  ExtrapMethod=Clip  InternalRulePriority=Speed  RndMeth=Simplest  InputSameDT=on
      settings: InputPortMap=u0,u1
  Product : Product  Inputs=**
  Crmbetad : Outport
  wires:
  CRMBDH_ALFA_M/1 -> Product/1
  angleOfAttack_deg/1 -> CRMBDH_ALFA_M/2
  mach_nd/1 -> CRMBDH_ALFA_M/1
  Product/1 -> Crmbetad/1
  betad/1 -> Product/2

== system kamerol/Aerodynamics/RollMomentCoefficient/MachRegion3/Crmblg/Crmblg_ ==
  dLG : Inport
  angleOfAttack_deg : Inport  Port=2
  angleOfSideslip_deg : Inport  Port=3
  CRMBLST_NG_DOOR_ALFA : Lookup_n-D  BreakpointsForDimension1=admireDB.aerodata_asym_ext.CRMBLST.breakpoints.ALFA  BreakpointsForDimension2=admireDB.aerodata_asym_ext.CRMBLST.breakpoints.NG_DOOR  BreakpointsForDimension3=[5, 7]  Table=admireDB.aerodata_asym_ext.CRMBLST.newTable  ExtrapMethod=Clip  InternalRulePriority=Speed  RndMeth=Simplest  InputSameDT=on
      settings: InputPortMap=u0,u1
  Degrees to Radians : simulink_extras/Transformations/Degrees to Radians
  Product : Product  Inputs=3
  Crmblg : Outport
  wires:
  Degrees to Radians/1 -> Product/3
  CRMBLST_NG_DOOR_ALFA/1 -> Product/2
  dLG/1 -> CRMBLST_NG_DOOR_ALFA/2, Product/1
  angleOfAttack_deg/1 -> CRMBLST_NG_DOOR_ALFA/1
  Product/1 -> Crmblg/1
  angleOfSideslip_deg/1 -> Degrees to Radians/1

== system kamerol/Aerodynamics/RollMomentCoefficient/MachRegion3/Crmdai/Crmdai_ ==
  angleOfAttack_deg : Inport
  dAI : Inport  Port=2
  mach_nd : Inport  Port=3
  dEI : Inport  Port=4
  eieff : Inport  Port=5
  qacorr : Inport  Port=6
  Abs : Abs
  CRMDA_ALFA_DE_M : Lookup_n-D  NumberOfTableDimensions=3  BreakpointsForDimension1=admireDB.aerodata_asym_ext.CRMDA.breakpoints.ALFA  BreakpointsForDimension2=admireDB.aerodata_asym_ext.CRMDA.breakpoints.DE  BreakpointsForDimension3=admireDB.aerodata_asym_ext.CRMDA.breakpoints.M  Table=admireDB.aerodata_asym_ext.CRMDA.newTable  ExtrapMethod=Clip  InternalRulePriority=Speed  RndMeth=Simplest  InputSameDT=on
      settings: InputPortMap=u0,u1,u2
  CRMDA_ALFA_DE_M1 : Lookup_n-D  NumberOfTableDimensions=3  BreakpointsForDimension1=admireDB.aerodata_asym_ext.CRMDA.breakpoints.ALFA  BreakpointsForDimension2=admireDB.aerodata_asym_ext.CRMDA.breakpoints.DE  BreakpointsForDimension3=admireDB.aerodata_asym_ext.CRMDA.breakpoints.M  Table=admireDB.aerodata_asym_ext.CRMDA.newTable  ExtrapMethod=Clip  InternalRulePriority=Speed  RndMeth=Simplest  InputSameDT=on
      settings: InputPortMap=u0,u1,u2
  CRMEDAI_QA_M : Lookup_n-D  BreakpointsForDimension1=admireDB.aerodata_asym_ext.CRMEDAI.breakpoints.M  BreakpointsForDimension2=admireDB.aerodata_asym_ext.CRMEDAI.breakpoints.QA  BreakpointsForDimension3=[5, 7]  Table=admireDB.aerodata_asym_ext.CRMEDAI.newTable  ExtrapMethod=Clip  InternalRulePriority=Speed  RndMeth=Simplest  InputSameDT=on
      settings: InputPortMap=u0,u1
  CRMMDAA_ALFA_DA_M : Lookup_n-D  NumberOfTableDimensions=3  BreakpointsForDimension1=admireDB.aerodata_asym_ext.CRMMDAA.breakpoints.ALFA  BreakpointsForDimension2=admireDB.aerodata_asym_ext.CRMMDAA.breakpoints.DA  BreakpointsForDimension3=admireDB.aerodata_asym_ext.CRMMDAA.breakpoints.M  Table=admireDB.aerodata_asym_ext.CRMMDAA.newTable  ExtrapMethod=Clip  InternalRulePriority=Speed  RndMeth=Simplest  InputSameDT=on
      settings: InputPortMap=u0,u1,u2
  Constant : Constant  Value=0
  Degrees to Radians : simulink_extras/Transformations/Degrees to Radians
  Product : Product  Inputs=**
  Product1 : Product
  Product3 : Product  Inputs=***
  Sign : Signum
  Sum : Sum  Inputs=|+-
  Sum1 : Sum  Inputs=|++
  Crmdai : Outport
  wires:
  Abs/1 -> CRMMDAA_ALFA_DA_M/2
  eieff/1 -> Product3/2
  qacorr/1 -> CRMEDAI_QA_M/2
  CRMEDAI_QA_M/1 -> Product3/3
  [mach] -> CRMEDAI_QA_M/1
  Product3/1 -> Crmdai/1
  Sum1/1 -> Product3/1
  Product1/1 -> Sum1/2
  Product/1 -> Sum1/1
  Degrees to Radians/1 -> Product1/1
  Sum/1 -> Product1/2
  [dAI] -> Sign/1, Degrees to Radians/1
  CRMDA_ALFA_DE_M1/1 -> Sum/2
  CRMDA_ALFA_DE_M/1 -> Sum/1
  Constant/1 -> CRMDA_ALFA_DE_M1/2
  dEI/1 -> CRMDA_ALFA_DE_M/2
  angleOfAttack_deg/1 -> CRMDA_ALFA_DE_M/1, CRMDA_ALFA_DE_M1/1, CRMMDAA_ALFA_DA_M/1
  mach_nd/1 -> [mach], CRMDA_ALFA_DE_M1/3, CRMDA_ALFA_DE_M/3, CRMMDAA_ALFA_DA_M/3
  dAI/1 -> [dAI], Abs/1
  Sign/1 -> Product/2
  CRMMDAA_ALFA_DA_M/1 -> Product/1

== system kamerol/Aerodynamics/RollMomentCoefficient/MachRegion3/Crmday/Crmday_ ==
  angleOfAttack_deg : Inport
  dAI : Inport  Port=2
  mach_nd : Inport  Port=3
  dEI : Inport  Port=4
  eieff : Inport  Port=5
  qacorr : Inport  Port=6
  Abs : Abs
  CRMDA_ALFA_DE_M : Lookup_n-D  NumberOfTableDimensions=3  BreakpointsForDimension1=admireDB.aerodata_asym_ext.CRMDA.breakpoints.ALFA  BreakpointsForDimension2=admireDB.aerodata_asym_ext.CRMDA.breakpoints.DE  BreakpointsForDimension3=admireDB.aerodata_asym_ext.CRMDA.breakpoints.M  Table=admireDB.aerodata_asym_ext.CRMDA.newTable  ExtrapMethod=Clip  InternalRulePriority=Speed  RndMeth=Simplest  InputSameDT=on
      settings: InputPortMap=u0,u1,u2
  CRMDA_ALFA_DE_M1 : Lookup_n-D  NumberOfTableDimensions=3  BreakpointsForDimension1=admireDB.aerodata_asym_ext.CRMDA.breakpoints.ALFA  BreakpointsForDimension2=admireDB.aerodata_asym_ext.CRMDA.breakpoints.DE  BreakpointsForDimension3=admireDB.aerodata_asym_ext.CRMDA.breakpoints.M  Table=admireDB.aerodata_asym_ext.CRMDA.newTable  ExtrapMethod=Clip  InternalRulePriority=Speed  RndMeth=Simplest  InputSameDT=on
      settings: InputPortMap=u0,u1,u2
  CRMEDAY_QA_M : Lookup_n-D  BreakpointsForDimension1=admireDB.aerodata_asym_ext.CRMEDAY.breakpoints.M  BreakpointsForDimension2=admireDB.aerodata_asym_ext.CRMEDAY.breakpoints.QA  BreakpointsForDimension3=[5, 7]  Table=admireDB.aerodata_asym_ext.CRMEDAY.newTable  ExtrapMethod=Clip  InternalRulePriority=Speed  RndMeth=Simplest  InputSameDT=on
      settings: InputPortMap=u0,u1
  CRMMDAA_ALFA_DA_M : Lookup_n-D  NumberOfTableDimensions=3  BreakpointsForDimension1=admireDB.aerodata_asym_ext.CRMMDAA.breakpoints.ALFA  BreakpointsForDimension2=admireDB.aerodata_asym_ext.CRMMDAA.breakpoints.DA  BreakpointsForDimension3=admireDB.aerodata_asym_ext.CRMMDAA.breakpoints.M  Table=admireDB.aerodata_asym_ext.CRMMDAA.newTable  ExtrapMethod=Clip  InternalRulePriority=Speed  RndMeth=Simplest  InputSameDT=on
      settings: InputPortMap=u0,u1,u2
  Constant : Constant  Value=0
  Degrees to Radians : simulink_extras/Transformations/Degrees to Radians
  Product : Product  Inputs=**
  Product1 : Product
  Product3 : Product  Inputs=***
  Sign : Signum
  Sum : Sum  Inputs=|+-
  Sum1 : Sum  Inputs=|++
  Crmdai : Outport
  wires:
  Abs/1 -> CRMMDAA_ALFA_DA_M/2
  eieff/1 -> Product3/2
  qacorr/1 -> CRMEDAY_QA_M/2
  CRMEDAY_QA_M/1 -> Product3/3
  [mach] -> CRMEDAY_QA_M/1
  Product3/1 -> Crmdai/1
  Sum1/1 -> Product3/1
  Product1/1 -> Sum1/2
  Product/1 -> Sum1/1
  Degrees to Radians/1 -> Product1/1
  Sum/1 -> Product1/2
  [dAI] -> Sign/1, Degrees to Radians/1
  CRMDA_ALFA_DE_M1/1 -> Sum/2
  CRMDA_ALFA_DE_M/1 -> Sum/1
  Constant/1 -> CRMDA_ALFA_DE_M1/2
  dEI/1 -> CRMDA_ALFA_DE_M/2
  angleOfAttack_deg/1 -> CRMDA_ALFA_DE_M/1, CRMDA_ALFA_DE_M1/1, CRMMDAA_ALFA_DA_M/1
  mach_nd/1 -> [mach], CRMDA_ALFA_DE_M1/3, CRMDA_ALFA_DE_M/3, CRMMDAA_ALFA_DA_M/3
  dAI/1 -> [dAI], Abs/1
  Sign/1 -> Product/2
  CRMMDAA_ALFA_DA_M/1 -> Product/1

== system kamerol/Aerodynamics/RollMomentCoefficient/MachRegion3/Crmdna/Crmdna_ ==
  angleOfAttack_deg : Inport
  dNA : Inport  Port=2
  CRMDNAAM_ALFA_M : Lookup_n-D  BreakpointsForDimension1=admireDB.aerodata_asym_ext.CRMDNAAM.breakpoints.M  BreakpointsForDimension2=admireDB.aerodata_asym_ext.CRMDNAAM.breakpoints.ALFA  BreakpointsForDimension3=[5, 7]  Table=admireDB.aerodata_asym_ext.CRMDNAAM.newTable  ExtrapMethod=Clip  InternalRulePriority=Speed  RndMeth=Simplest  InputSameDT=on
      settings: InputPortMap=u0,u1
  Degrees to Radians : simulink_extras/Transformations/Degrees to Radians
  Product : Product  Inputs=**
  mach_nd_cnst : Constant  Value=0.5
  Crmdna : Outport
  wires:
  Degrees to Radians/1 -> Product/2
  dNA/1 -> Degrees to Radians/1
  mach_nd_cnst/1 -> CRMDNAAM_ALFA_M/1
  Product/1 -> Crmdna/1
  angleOfAttack_deg/1 -> CRMDNAAM_ALFA_M/2
  CRMDNAAM_ALFA_M/1 -> Product/1

== system kamerol/Aerodynamics/RollMomentCoefficient/MachRegion3/Crmdr/Crmdr_ ==
  qacorr : Inport
  mach_nd : Inport  Port=2
  dR : Inport  Port=3
  CRMDRM_M : Lookup_n-D  NumberOfTableDimensions=1  BreakpointsForDimension1=admireDB.aerodata_asym_ext.CRMDRM.breakpoints.M  BreakpointsForDimension3=[5, 7]  Table=admireDB.aerodata_asym_ext.CRMDRM.newTable  ExtrapMethod=Clip  InternalRulePriority=Speed  RndMeth=Simplest  InputSameDT=on
  CRMEDR_QA_M : Lookup_n-D  BreakpointsForDimension1=admireDB.aerodata_asym_ext.CRMEDR.breakpoints.M  BreakpointsForDimension2=admireDB.aerodata_asym_ext.CRMEDR.breakpoints.QA  BreakpointsForDimension3=[5, 7]  Table=admireDB.aerodata_asym_ext.CRMEDR.newTable  ExtrapMethod=Clip  InternalRulePriority=Speed  RndMeth=Simplest  InputSameDT=on
      settings: InputPortMap=u0,u1
  Degrees to Radians : simulink_extras/Transformations/Degrees to Radians
  Product2 : Product  Inputs=3
  Crmdr : Outport
  wires:
  dR/1 -> Degrees to Radians/1
  CRMDRM_M/1 -> Product2/1
  Degrees to Radians/1 -> Product2/2
  qacorr/1 -> CRMEDR_QA_M/2
  mach_nd/1 -> CRMEDR_QA_M/1, CRMDRM_M/1
  CRMEDR_QA_M/1 -> Product2/3
  Product2/1 -> Crmdr/1

== system kamerol/Aerodynamics/RollMomentCoefficient/MachRegion3/Crmp/Crmp_ ==
  angleOfAttack_deg : Inport
  mach_nd : Inport  Port=2
  pc : Inport  Port=3
  qacorr : Inport  Port=4
  CRMEP_QA_M : Lookup_n-D  BreakpointsForDimension1=admireDB.aerodata_asym_ext.CRMEP.breakpoints.M  BreakpointsForDimension2=admireDB.aerodata_asym_ext.CRMEP.breakpoints.QA  BreakpointsForDimension3=[5, 7]  Table=admireDB.aerodata_asym_ext.CRMEP.newTable  ExtrapMethod=Clip  InternalRulePriority=Speed  RndMeth=Simplest  InputSameDT=on
      settings: InputPortMap=u0,u1
  CRMPAM_ALFA_M : Lookup_n-D  BreakpointsForDimension1=admireDB.aerodata_asym_ext.CRMPAM.breakpoints.M  BreakpointsForDimension2=admireDB.aerodata_asym_ext.CRMPAM.breakpoints.ALFA  BreakpointsForDimension3=[5, 7]  Table=admireDB.aerodata_asym_ext.CRMPAM.newTable  ExtrapMethod=Clip  InternalRulePriority=Speed  RndMeth=Simplest  InputSameDT=on
      settings: InputPortMap=u0,u1
  Product : Product  Inputs=3
  Crmp : Outport
  wires:
  qacorr/1 -> CRMEP_QA_M/2
  CRMPAM_ALFA_M/1 -> Product/1
  angleOfAttack_deg/1 -> CRMPAM_ALFA_M/2
  Product/1 -> Crmp/1
  pc/1 -> Product/2
  CRMEP_QA_M/1 -> Product/3
  mach_nd/1 -> CRMPAM_ALFA_M/1, CRMEP_QA_M/1

== system kamerol/Aerodynamics/RollMomentCoefficient/MachRegion3/Crmr/Crmr_ ==
  angleOfAttack_deg : Inport
  mach_nd : Inport  Port=2
  rc : Inport  Port=3
  CRMRAM_ALFA_M : Lookup_n-D  BreakpointsForDimension1=admireDB.aerodata_asym_ext.CRMRAM.breakpoints.M  BreakpointsForDimension2=admireDB.aerodata_asym_ext.CRMRAM.breakpoints.ALFA  BreakpointsForDimension3=[5, 7]  Table=admireDB.aerodata_asym_ext.CRMRAM.newTable  ExtrapMethod=Clip  InternalRulePriority=Speed  RndMeth=Simplest  InputSameDT=on
      settings: InputPortMap=u0,u1
  Product : Product  Inputs=**
  Crmr : Outport
  wires:
  CRMRAM_ALFA_M/1 -> Product/1
  mach_nd/1 -> CRMRAM_ALFA_M/1
  angleOfAttack_deg/1 -> CRMRAM_ALFA_M/2
  Product/1 -> Crmr/1
  rc/1 -> Product/2

== system kamerol/Aerodynamics/RollMomentCoefficient/MachRegion3/Crmrde/Crmrde_ ==
  mach_nd : Inport
  angleOfAttack_deg : Inport  Port=2
  rc : Inport  Port=3
  dEI : Inport  Port=4
  eieff : Inport  Port=5
  dEY : Inport  Port=6
  eoeff : Inport  Port=7
  CRMRDEM_M : Lookup_n-D  NumberOfTableDimensions=1  BreakpointsForDimension1=admireDB.aerodata_asym_ext.CRMRDEM.breakpoints.M  BreakpointsForDimension3=[5, 7]  Table=admireDB.aerodata_asym_ext.CRMRDEM.newTable  ExtrapMethod=Clip  InternalRulePriority=Speed  RndMeth=Simplest  InputSameDT=on
  CRMRKA_ALFA : Lookup_n-D  NumberOfTableDimensions=1  BreakpointsForDimension1=admireDB.aerodata_asym_ext.CRMRKA.breakpoints.ALFA  BreakpointsForDimension3=[5, 7]  Table=admireDB.aerodata_asym_ext.CRMRKA.newTable  ExtrapMethod=Clip  InternalRulePriority=Speed  RndMeth=Simplest  InputSameDT=on
  Constant : Constant  Value=1/30
  Constant1 : Constant  Value=1/30
  Product : Product  Inputs=****
  Product1 : Product  Inputs=3
  Product2 : Product  Inputs=3
  Sum : Sum  Inputs=|++
  Crmrde : Outport
  wires:
  Sum/1 -> Product/4
  Product2/1 -> Sum/2
  Product1/1 -> Sum/1
  dEY/1 -> Product2/1
  eoeff/1 -> Product2/3
  Constant1/1 -> Product2/2
  Constant/1 -> Product1/2
  eieff/1 -> Product1/3
  dEI/1 -> Product1/1
  CRMRKA_ALFA/1 -> Product/2
  CRMRDEM_M/1 -> Product/1
  mach_nd/1 -> CRMRDEM_M/1
  angleOfAttack_deg/1 -> CRMRKA_ALFA/1
  Product/1 -> Crmrde/1
  rc/1 -> Product/3

== system kamerol/Aerodynamics/RollMomentCoefficient/MachRegion4/Crmbde/Crmbde_ ==
  angleOfAttack_deg : Inport
  dN : Inport  Port=2
  dEI : Inport  Port=3
  angleOfSideslip_deg : Inport  Port=4
  dEY : Inport  Port=5
  eieff : Inport  Port=6
  eoeff : Inport  Port=7
  mach_nd : Inport  Port=8
  Abs : Abs
  CRMBKM_M : Lookup_n-D  NumberOfTableDimensions=1  BreakpointsForDimension1=admireDB.aerodata_asym_ext.CRMBKM.breakpoints.M  BreakpointsForDimension3=[5, 7]  Table=admireDB.aerodata_asym_ext.CRMBKM.newTable  ExtrapMethod=Clip  InternalRulePriority=Speed  RndMeth=Simplest  InputSameDT=on
  CRMDEB_ALFA_DN_DE_BETA : Lookup_n-D  NumberOfTableDimensions=4  BreakpointsForDimension1=admireDB.aerodata_asym_ext.CRMDEB.breakpoints.ALFA  BreakpointsForDimension2=admireDB.aerodata_asym_ext.CRMDEB.breakpoints.DN  BreakpointsForDimension3=admireDB.aerodata_asym_ext.CRMDEB.breakpoints.DE  BreakpointsForDimension4=admireDB.aerodata_asym_ext.CRMDEB.breakpoints.BETA  Table=admireDB.aerodata_asym_ext.CRMDEB.newTable  ExtrapMethod=Clip  InternalRulePriority=Speed  RndMeth=Simplest  InputSameDT=on
      settings: InputPortMap=u0,u1,u2,u3
  CRMDEB_ALFA_DN_DE_BETA1 : Lookup_n-D  NumberOfTableDimensions=4  BreakpointsForDimension1=admireDB.aerodata_asym_ext.CRMDEB.breakpoints.ALFA  BreakpointsForDimension2=admireDB.aerodata_asym_ext.CRMDEB.breakpoints.DN  BreakpointsForDimension3=admireDB.aerodata_asym_ext.CRMDEB.breakpoints.DE  BreakpointsForDimension4=admireDB.aerodata_asym_ext.CRMDEB.breakpoints.BETA  Table=admireDB.aerodata_asym_ext.CRMDEB.newTable  ExtrapMethod=Clip  InternalRulePriority=Speed  RndMeth=Simplest  InputSameDT=on
      settings: InputPortMap=u0,u1,u2,u3
  Product : Product  Inputs=**
  Product1 : Product  Inputs=**
  Product2 : Product  Inputs=3
  Sign : Signum
  Sum : Sum  Inputs=|++
  Crmbde : Outport
  wires:
  dEY/1 -> CRMDEB_ALFA_DN_DE_BETA1/3
  angleOfAttack_deg/1 -> CRMDEB_ALFA_DN_DE_BETA1/1, CRMDEB_ALFA_DN_DE_BETA/1
  dN/1 -> CRMDEB_ALFA_DN_DE_BETA/2, CRMDEB_ALFA_DN_DE_BETA1/2
  dEI/1 -> CRMDEB_ALFA_DN_DE_BETA/3
  Abs/1 -> CRMDEB_ALFA_DN_DE_BETA/4, CRMDEB_ALFA_DN_DE_BETA1/4
  CRMBKM_M/1 -> Product2/3
  mach_nd/1 -> CRMBKM_M/1
  Sign/1 -> Product2/1
  Product2/1 -> Crmbde/1
  Product1/1 -> Sum/2
  Product/1 -> Sum/1
  Sum/1 -> Product2/2
  eoeff/1 -> Product1/1
  eieff/1 -> Product/2
  CRMDEB_ALFA_DN_DE_BETA1/1 -> Product1/2
  CRMDEB_ALFA_DN_DE_BETA/1 -> Product/1
  angleOfSideslip_deg/1 -> Sign/1, Abs/1

== system kamerol/Aerodynamics/RollMomentCoefficient/MachRegion4/Crmbdle/Crmbdle_ ==
  angleOfAttack_deg : Inport
  dEI : Inport  Port=2
  mach_nd : Inport  Port=3
  dEY : Inport  Port=4
  eieff : Inport  Port=5
  eoeff : Inport  Port=6
  angleOfSideslip_deg : Inport  Port=7
  dLE : Inport  Port=8
  CRMBDLE_ALFA_DE_M : Lookup_n-D  NumberOfTableDimensions=3  BreakpointsForDimension1=admireDB.aerodata_asym_ext.CRMBDLE.breakpoints.ALFA  BreakpointsForDimension2=admireDB.aerodata_asym_ext.CRMBDLE.breakpoints.DE  BreakpointsForDimension3=admireDB.aerodata_asym_ext.CRMBDLE.breakpoints.M  Table=admireDB.aerodata_asym_ext.CRMBDLE.newTable  ExtrapMethod=Clip  InternalRulePriority=Speed  RndMeth=Simplest  InputSameDT=on
      settings: InputPortMap=u0,u1,u2
  CRMBDLE_ALFA_DE_M1 : Lookup_n-D  NumberOfTableDimensions=3  BreakpointsForDimension1=admireDB.aerodata_asym_ext.CRMBDLE.breakpoints.ALFA  BreakpointsForDimension2=admireDB.aerodata_asym_ext.CRMBDLE.breakpoints.DE  BreakpointsForDimension3=admireDB.aerodata_asym_ext.CRMBDLE.breakpoints.M  Table=admireDB.aerodata_asym_ext.CRMBDLE.newTable  ExtrapMethod=Clip  InternalRulePriority=Speed  RndMeth=Simplest  InputSameDT=on
      settings: InputPortMap=u0,u1,u2
  Constant : Constant  Value=1/27
  Degrees to Radians : simulink_extras/Transformations/Degrees to Radians
  Product : Product  Inputs=**
  Product1 : Product  Inputs=**
  Product2 : Product  Inputs=****
  Sum : Sum  Inputs=|++
  Crmbdle : Outport
  wires:
  dEY/1 -> CRMBDLE_ALFA_DE_M1/2
  dEI/1 -> CRMBDLE_ALFA_DE_M/2
  mach_nd/1 -> CRMBDLE_ALFA_DE_M/3, CRMBDLE_ALFA_DE_M1/3
  angleOfAttack_deg/1 -> CRMBDLE_ALFA_DE_M/1, CRMBDLE_ALFA_DE_M1/1
  Product2/1 -> Crmbdle/1
  Constant/1 -> Product2/4
  Sum/1 -> Product2/2
  Product1/1 -> Sum/2
  Product/1 -> Sum/1
  dLE/1 -> Product2/3
  Degrees to Radians/1 -> Product2/1
  angleOfSideslip_deg/1 -> Degrees to Radians/1
  CRMBDLE_ALFA_DE_M1/1 -> Product1/1
  eoeff/1 -> Product1/2
  CRMBDLE_ALFA_DE_M/1 -> Product/1
  eieff/1 -> Product/2

== system kamerol/Aerodynamics/RollMomentCoefficient/MachRegion4/Crmbdn/Crmbdn_ ==
  dN : Inport
  mach_nd : Inport  Port=2
  angleOfSideslip_deg : Inport  Port=3
  CRMBMDN_DN_M : Lookup_n-D  BreakpointsForDimension1=admireDB.aerodata_asym_ext.CRMBMDN.breakpoints.M  BreakpointsForDimension2=admireDB.aerodata_asym_ext.CRMBMDN.breakpoints.DN  BreakpointsForDimension3=[5, 7]  Table=admireDB.aerodata_asym_ext.CRMBMDN.newTable  ExtrapMethod=Clip  InternalRulePriority=Speed  RndMeth=Simplest  InputSameDT=on
      settings: InputPortMap=u0,u1
  Degrees to Radians : simulink_extras/Transformations/Degrees to Radians
  Product : Product  Inputs=**
  Crmbdn : Outport
  wires:
  Product/1 -> Crmbdn/1
  CRMBMDN_DN_M/1 -> Product/1
  angleOfSideslip_deg/1 -> Degrees to Radians/1
  mach_nd/1 -> CRMBMDN_DN_M/1
  Degrees to Radians/1 -> Product/2
  dN/1 -> CRMBMDN_DN_M/2

== system kamerol/Aerodynamics/RollMomentCoefficient/MachRegion4/Crmbeta/Crmbeta_ ==
  mach_nd : Inport
  angleOfAttack_deg : Inport  Port=2
  angleOfSideslip_deg : Inport  Port=3
  qacorr : Inport  Port=4
  CRMBMA_M_ALFA : Lookup_n-D  BreakpointsForDimension1=admireDB.aerodata_asym_ext.CRMBMA.breakpoints.ALFA  BreakpointsForDimension2=admireDB.aerodata_asym_ext.CRMBMA.breakpoints.M  BreakpointsForDimension3=[5, 7]  Table=admireDB.aerodata_asym_ext.CRMBMA.newTable  ExtrapMethod=Clip  InternalRulePriority=Speed  RndMeth=Simplest  InputSameDT=on
      settings: InputPortMap=u0,u1
  CRMEB_QA_M : Lookup_n-D  BreakpointsForDimension1=admireDB.aerodata_asym_ext.CRMEB.breakpoints.M  BreakpointsForDimension2=admireDB.aerodata_asym_ext.CRMEB.breakpoints.QA  BreakpointsForDimension3=[5, 7]  Table=admireDB.aerodata_asym_ext.CRMEB.newTable  ExtrapMethod=Clip  InternalRulePriority=Speed  RndMeth=Simplest  InputSameDT=on
      settings: InputPortMap=u0,u1
  Degrees to Radians : simulink_extras/Transformations/Degrees to Radians
  Product1 : Product
  Sum : Sum  Inputs=|++
  Crmbeta : Outport
  wires:
  CRMBMA_M_ALFA/1 -> Sum/1
  mach_nd/1 -> CRMBMA_M_ALFA/2, CRMEB_QA_M/1
  angleOfAttack_deg/1 -> CRMBMA_M_ALFA/1
  qacorr/1 -> CRMEB_QA_M/2
  angleOfSideslip_deg/1 -> Degrees to Radians/1
  CRMEB_QA_M/1 -> Product1/2
  Degrees to Radians/1 -> Product1/1
  Product1/1 -> Sum/2
  Sum/1 -> Crmbeta/1
